simulink model "math_int_3_test"  (Simulink 7.2)
settings: Solver=VariableStepDiscrete  StartTime=0.0  StopTime=10.0  RelTol=1e-3
settings Model: Creator=arnaud  LastModifiedBy=arnaud
settings DataIOCC: SaveFormat=Structure

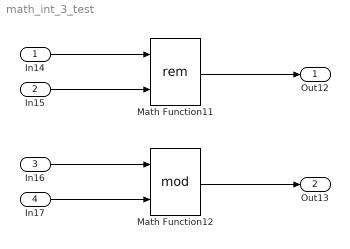
== system math_int_3_test ==
  In14 : Inport  DataType=int8  OutDataType=sfix(16)  OutScaling=2^0  OutDataTypeStr=int8
  In15 : Inport  Port=2  DataType=int8  OutDataType=sfix(16)  OutScaling=2^0  OutDataTypeStr=int8
  In16 : Inport  Port=3  DataType=int8  OutDataType=sfix(16)  OutScaling=2^0  OutDataTypeStr=int8
  In17 : Inport  Port=4  DataType=int8  OutDataType=sfix(16)  OutScaling=2^0  OutDataTypeStr=int8
  Math Function11 : Math  Operator=rem  OutDataType=sfix(16)  OutScaling=2^0  SaturateOnIntegerOverflow=on
  Math Function12 : Math  Operator=mod  OutDataType=sfix(16)  OutScaling=2^0  SaturateOnIntegerOverflow=on
  Out12 : Outport  OutDataType=sfix(16)  OutScaling=2^0
  Out13 : Outport  Port=2  OutDataType=sfix(16)  OutScaling=2^0
  wires:
  In14/1 -> Math Function11/1
  In15/1 -> Math Function11/2
  Math Function11/1 -> Out12/1
  In16/1 -> Math Function12/1
  In17/1 -> Math Function12/2
  Math Function12/1 -> Out13/1
